simulink model "slexModelingServicesExample"  (R2019b)
settings: Solver=FixedStepAuto  StartTime=0.0  StopTime=10.0  RelTol=1e-3  EnableMultiTasking=on
settings Model: Creator=The MathWorks, Inc.  LastModifiedBy=bhisma
settings SolverCC: PositivePriorityOrder=on
settings DataIOCC: SaveFormat=StructureWithTime
settings OptimizationCC: DefaultParameterBehavior=Inlined  PassReuseOutputArgsAs=Individual arguments  MaxStackSize=64  EfficientTunableParamExpr=on
settings DebuggingCC: ParameterTunabilityLossMsg=error  ArithmeticOperatorsInVariantConditions=warning
settings HardwareCC: ProdBitPerPointer=32  ProdBitPerSizeT=32  ProdBitPerPtrDiffT=32  ProdLargestAtomicInteger=Long  ProdLargestAtomicFloat=Double  ProdWordSize=32  ProdHWDeviceType=ARM Compatible->ARM Cortex
settings SFSimCC: SimUseLocalCustomCode=off  MATLABDynamicMemAlloc=off  CustomCodeUndefinedFunction=UseInterfaceOnly
settings RTWCC: SystemTargetFile=ert.tlc  TemplateMakefile=ert_default_tmf  GenerateReport=on  RTWUseLocalCustomCode=off  IncludeHyperlinkInReport=on  LaunchReport=on  GenerateTraceInfo=on  GenerateTraceReport=on  GenerateTraceReportSl=on  GenerateTraceReportSf=on  GenerateTraceReportEml=on
settings CodeAppCC: ForceParamTrailComments=on  IgnoreCustomStorageClasses=off  MaxIdLength=63  OperatorAnnotations=on  SimulinkDataObjDesc=on  SFDataObjDesc=on  InsertBlockDesc=on
settings ERTTargetCC: SupportVariableSizeSignals=on  ERTCustomFileTemplate=example_file_process.tlc

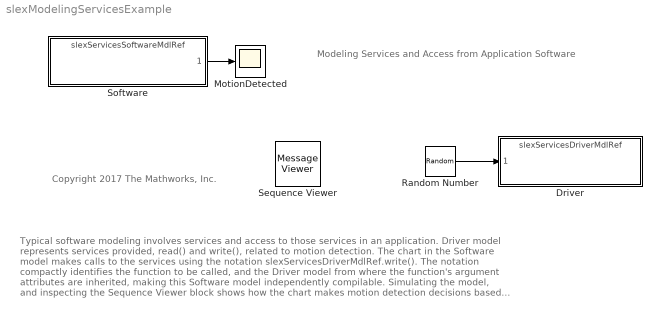
== system slexModelingServicesExample ==
  note: Modeling Services and Access from Application Software
  note: Copyright 2017 The Mathworks, Inc.
  note: Typical software modeling involves services and access to those services in an application. Driver model represents services provided, read() and write(), related to motion detection.
      |
      | The chart in the Software model makes calls to the services using the notation slexServicesDriverMdlRef.write(). The notation compactly identifies the function to be called, and the Driver model from where the function's argument attributes are inherited, making this Software model independently compilable.
      |
      | Simulating the model, and inspecting the Sequence Viewer block shows how the chart makes motion detection decisions based on the services.
  Driver : ModelReference  ModelNameDialog=slexServicesDriverMdlRef.slx  SimulationMode=Normal  ScheduleRates=on  ModelReferenceVersion=1.42
  MotionDetected : Scope
  Random Number : RandomNumber  SampleTime=0.1
  Sequence Viewer : MessageViewer
  Software : ModelReference  ModelNameDialog=slexServicesSoftwareMdlRef.slx  SimulationMode=Normal  ModelReferenceVersion=1.35
  wires:
  Random Number/1 -> Driver/1
  Software/1 -> MotionDetected/1
